simulink model "SimParking"  (R2017b)
settings: Solver=VariableStepAuto  StartTime=0.0  StopTime=1761  RelTol=1e-3
libraries: neural x1111
(part 51 of 60)

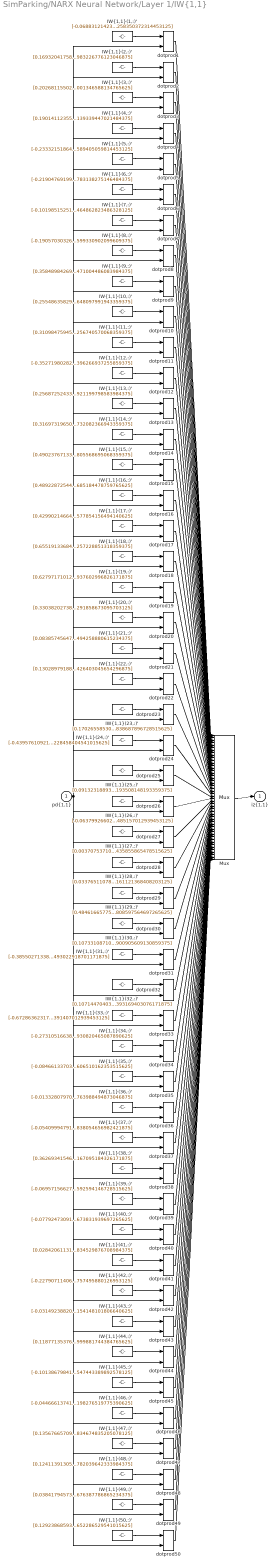
== system SimParking/NARX Neural Network/Layer 1/IW{1,1} ==
  "pd{1,1}" : Inport  PortDimensions=9  SampleTime=1
      mask Display: e = 0.06;c1 = [120 230 180]/255;c2 = ([120 230 180]+0)/(256+128);c3 = ([120 230 180]+128)/(256+128);patch([0 1 1 0],[0 0 1 1],c1);patch([0 1 1 1-e 1-e 0+e],[0 0 1 1-e 0+e 0+e],c2);patch([0 0 1 1-e 0+e 0+e],[0 1 1 1-e 1-e 0+e],c3);plot([0 1 1 0 0],[0 0 1 1 0]);
  "IW{1,1}(1,:)'" : Constant  Value=[-0.0688312142351427402875430061612860299646854400634765625;-0.00731147282474513271477434273037943057715892791748046875;0.264160400589513566504962227554642595350742340087890625;-0.2702584075688310161211802551406435668468475341796875;-0.256440287705181180211155833603697828948497772216796875;-0.032637463492422490174416083164032897911965847015380859375;0.0715212296441626038667749298838316462934017181396484375;-0.2454744006920569765473061352167860604822635650634765625;0.1741091167626269697876750797149725258350372314453125]
      mask Display: e = 0.06;c1 = [120 150 230]/255;c2 = ([120 150 230]+0)/383;c3 = ([120 150 230]+128)/383;patch([0 1 1 0],[0 0 1 1],c1);patch([0 1 1 1-e 1-e 0+e],[0 0 1 1-e 0+e 0+e],c2);patch([0 0 1 1-e 0+e 0+e],[0 1 1 1-e 1-e 0+e],c3);plot([0 1 1 0 0],[0 0 1 1 0]);disp('Weights');
  "IW{1,1}(10,:)'" : Constant  Value=[0.2554863582900424034960451535880565643310546875;0.0958506165966647449838688999079749919474124908447265625;-0.32565209786216886556076133274473249912261962890625;0.30664766510793473042184587029623799026012420654296875;0.045108980545902059577922926791870850138366222381591796875;0.13081971515873325184742270721471868455410003662109375;0.30795940572873325979941228069947101175785064697265625;0.023228248459151619453866288722565514035522937774658203125;0.2355814180893774645308980097979656420648097991943359375]
      mask Display: e = 0.06;c1 = [120 150 230]/255;c2 = ([120 150 230]+0)/383;c3 = ([120 150 230]+128)/383;patch([0 1 1 0],[0 0 1 1],c1);patch([0 1 1 1-e 1-e 0+e],[0 0 1 1-e 0+e 0+e],c2);patch([0 0 1 1-e 0+e 0+e],[0 1 1 1-e 1-e 0+e],c3);plot([0 1 1 0 0],[0 0 1 1 0]);disp('Weights');
  "IW{1,1}(11,:)'" : Constant  Value=[0.3109847594544794535664777868078090250492095947265625;-0.285941876296102959198464077417156659066677093505859375;-0.03748334600944412675627148701096302829682826995849609375;-0.4303286602511013914096338339732028543949127197265625;-0.2985573957135070344293126254342496395111083984375;0.82416954716962342875063995961681939661502838134765625;0.1697649234253264249883130787566187791526317596435546875;0.06921903233537364530381097438294091261923313140869140625;-0.27516488517038906191913838483742438256740570068359375]
      mask Display: e = 0.06;c1 = [120 150 230]/255;c2 = ([120 150 230]+0)/383;c3 = ([120 150 230]+128)/383;patch([0 1 1 0],[0 0 1 1],c1);patch([0 1 1 1-e 1-e 0+e],[0 0 1 1-e 0+e 0+e],c2);patch([0 0 1 1-e 0+e 0+e],[0 1 1 1-e 1-e 0+e],c3);plot([0 1 1 0 0],[0 0 1 1 0]);disp('Weights');
  "IW{1,1}(12,:)'" : Constant  Value=[-0.352719802824051964496021582817775197327136993408203125;-0.069499098052672791947514951971243135631084442138671875;0.3030956741440811175181124781374819576740264892578125;-0.3374792645368049903709106729365885257720947265625;0.00816585423091213853663550281680727493949234485626220703125;-0.19962942893532698018788096305797807872295379638671875;-0.20286919149293736186479009120375849306583404541015625;-0.199431767288725747544475552786025218665599822998046875;-0.345388528908461223121406646896502934396266937255859375]
      mask Display: e = 0.06;c1 = [120 150 230]/255;c2 = ([120 150 230]+0)/383;c3 = ([120 150 230]+128)/383;patch([0 1 1 0],[0 0 1 1],c1);patch([0 1 1 1-e 1-e 0+e],[0 0 1 1-e 0+e 0+e],c2);patch([0 0 1 1-e 0+e 0+e],[0 1 1 1-e 1-e 0+e],c3);plot([0 1 1 0 0],[0 0 1 1 0]);disp('Weights');
  "IW{1,1}(13,:)'" : Constant  Value=[0.256872524336901164598856439624796621501445770263671875;0.21350569072795588798641119865351356565952301025390625;-0.418804132286997532474970284965820610523223876953125;0.056591801455811004128992891537563991732895374298095703125;-0.07494113318384544586425732859424897469580173492431640625;0.2407993622761351593108969382228679023683071136474609375;0.059849568133809205594531022143200971186161041259765625;-0.060497754657408787937189487138311960734426975250244140625;0.00676880576702837931379885816340902238152921199798583984375]
      mask Display: e = 0.06;c1 = [120 150 230]/255;c2 = ([120 150 230]+0)/383;c3 = ([120 150 230]+128)/383;patch([0 1 1 0],[0 0 1 1],c1);patch([0 1 1 1-e 1-e 0+e],[0 0 1 1-e 0+e 0+e],c2);patch([0 0 1 1-e 0+e 0+e],[0 1 1 1-e 1-e 0+e],c3);plot([0 1 1 0 0],[0 0 1 1 0]);disp('Weights');
  "IW{1,1}(14,:)'" : Constant  Value=[0.316973196504036158760442276616231538355350494384765625;0.3247560829361930689884729872574098408222198486328125;0.53408347016352852865139766436186619102954864501953125;1.58975198318718202727950483676977455615997314453125;0.02759094957294229433220067448928602971136569976806640625;0.52886285187823889319957970656105317175388336181640625;0.50574814490768116304053592102718539535999298095703125;0.1567072528818204413258996510194265283644199371337890625;0.45264913068915146876491917282692156732082366943359375]
      mask Display: e = 0.06;c1 = [120 150 230]/255;c2 = ([120 150 230]+0)/383;c3 = ([120 150 230]+128)/383;patch([0 1 1 0],[0 0 1 1],c1);patch([0 1 1 1-e 1-e 0+e],[0 0 1 1-e 0+e 0+e],c2);patch([0 0 1 1-e 0+e 0+e],[0 1 1 1-e 1-e 0+e],c3);plot([0 1 1 0 0],[0 0 1 1 0]);disp('Weights');
  "IW{1,1}(15,:)'" : Constant  Value=[0.490237671330177759987378749428899027407169342041015625;0.1653204385555413491459830765961669385433197021484375;-0.79290809621698421505442411216790787875652313232421875;-0.56394479296315769278891139038023538887500762939453125;-0.01259539013756067089844226103423352469690144062042236328125;0.120847701090714354510424755062558688223361968994140625;0.11626089019634051890950132701618713326752185821533203125;0.52967211475309439183689619312644936144351959228515625;0.0275738220937100896035243380310930660925805568695068359375]
      mask Display: e = 0.06;c1 = [120 150 230]/255;c2 = ([120 150 230]+0)/383;c3 = ([120 150 230]+128)/383;patch([0 1 1 0],[0 0 1 1],c1);patch([0 1 1 1-e 1-e 0+e],[0 0 1 1-e 0+e 0+e],c2);patch([0 0 1 1-e 0+e 0+e],[0 1 1 1-e 1-e 0+e],c3);plot([0 1 1 0 0],[0 0 1 1 0]);disp('Weights');
  "IW{1,1}(16,:)'" : Constant  Value=[0.489228725449045998008301694426336325705051422119140625;-0.12693905925192827677250306805945001542568206787109375;0.1444743099035981914735060627208440564572811126708984375;0.43394957527358801741002025664784014225006103515625;0.1301043144415301444638544126064516603946685791015625;0.185288074364715560360394874805933795869350433349609375;0.3632901734391797976542193282512016594409942626953125;0.272778700473264190673461371261510066688060760498046875;0.0155539985865831321965035982657354907132685184478759765625]
      mask Display: e = 0.06;c1 = [120 150 230]/255;c2 = ([120 150 230]+0)/383;c3 = ([120 150 230]+128)/383;patch([0 1 1 0],[0 0 1 1],c1);patch([0 1 1 1-e 1-e 0+e],[0 0 1 1-e 0+e 0+e],c2);patch([0 0 1 1-e 0+e 0+e],[0 1 1 1-e 1-e 0+e],c3);plot([0 1 1 0 0],[0 0 1 1 0]);disp('Weights');
  "IW{1,1}(17,:)'" : Constant  Value=[0.429902146643838689588079660097719170153141021728515625;0.257765727905190866753315503956400789320468902587890625;-0.1500747886843795397826539783636690117418766021728515625;0.278788719014294417153365657213726080954074859619140625;0.276750512007699234207080962733016349375247955322265625;-0.82138062848648729641354293562471866607666015625;0.27536313592640848657566721158218570053577423095703125;0.1430395985820490933893012197586358524858951568603515625;0.348188489253207722473604235347011126577854156494140625]
      mask Display: e = 0.06;c1 = [120 150 230]/255;c2 = ([120 150 230]+0)/383;c3 = ([120 150 230]+128)/383;patch([0 1 1 0],[0 0 1 1],c1);patch([0 1 1 1-e 1-e 0+e],[0 0 1 1-e 0+e 0+e],c2);patch([0 0 1 1-e 0+e 0+e],[0 1 1 1-e 1-e 0+e],c3);plot([0 1 1 0 0],[0 0 1 1 0]);disp('Weights');
  "IW{1,1}(18,:)'" : Constant  Value=[0.65519133684555008745320492380415089428424835205078125;-0.456854910966180527420732460086583159863948822021484375;1.3571548324974906929440976455225609242916107177734375;0.34003096030817392403378107701428234577178955078125;-0.29173479660044321359890773237566463649272918701171875;0.376176211592635867386746895135729573667049407958984375;0.234861025309017090734187149791978299617767333984375;0.320971922147644417311340703236055560410022735595703125;0.1188667057288495809697081995182088576257228851318359375]
      mask Display: e = 0.06;c1 = [120 150 230]/255;c2 = ([120 150 230]+0)/383;c3 = ([120 150 230]+128)/383;patch([0 1 1 0],[0 0 1 1],c1);patch([0 1 1 1-e 1-e 0+e],[0 0 1 1-e 0+e 0+e],c2);patch([0 0 1 1-e 0+e 0+e],[0 1 1 1-e 1-e 0+e],c3);plot([0 1 1 0 0],[0 0 1 1 0]);disp('Weights');
  "IW{1,1}(19,:)'" : Constant  Value=[0.6279717101208761587116669034003280103206634521484375;-0.215597262533756051094968597681145183742046356201171875;-0.62907101345034532879907374081085436046123504638671875;-0.495109753658072804238798880760441534221172332763671875;-0.05778022558784827455991006672775256447494029998779296875;-1.0225979740194868217173507218831218779087066650390625;-0.03403932971557062370226987013666075654327869415283203125;-0.30098566072865640119715635592001490294933319091796875;-0.0220281334301075486237220246721335570327937602996826171875]
      mask Display: e = 0.06;c1 = [120 150 230]/255;c2 = ([120 150 230]+0)/383;c3 = ([120 150 230]+128)/383;patch([0 1 1 0],[0 0 1 1],c1);patch([0 1 1 1-e 1-e 0+e],[0 0 1 1-e 0+e 0+e],c2);patch([0 0 1 1-e 0+e 0+e],[0 1 1 1-e 1-e 0+e],c3);plot([0 1 1 0 0],[0 0 1 1 0]);disp('Weights');
  "IW{1,1}(2,:)'" : Constant  Value=[0.1693204175805965994161539356355206109583377838134765625;-0.280434391905482416351702568135806359350681304931640625;0.5574414461071182103069077129475772380828857421875;0.1491102386444250471608796715372591279447078704833984375;-0.139621185316120388630878323965589515864849090576171875;0.413097455057599594052675229249871335923671722412109375;-0.0987573011740672523917083935884875245392322540283203125;0.285585829665227441953589959666715003550052642822265625;0.09414021440129786977291104221876594237983226776123046875]
      mask Display: e = 0.06;c1 = [120 150 230]/255;c2 = ([120 150 230]+0)/383;c3 = ([120 150 230]+128)/383;patch([0 1 1 0],[0 0 1 1],c1);patch([0 1 1 1-e 1-e 0+e],[0 0 1 1-e 0+e 0+e],c2);patch([0 0 1 1-e 0+e 0+e],[0 1 1 1-e 1-e 0+e],c3);plot([0 1 1 0 0],[0 0 1 1 0]);disp('Weights');
  "IW{1,1}(20,:)'" : Constant  Value=[0.3303820273860218481587480710004456341266632080078125;0.042681097483308734485962787630342063494026660919189453125;-4.19220558490714179100677938549779355525970458984375;-2.64104506999998900340642649098299443721771240234375;0.124710532719106648169571371909114532172679901123046875;-0.20265695712461428978912181264604441821575164794921875;0.2237739206169422623293741025918279774487018585205078125;0.263060219041964693520441187502001412212848663330078125;0.72859097760744984118019829111290164291858673095703125]
      mask Display: e = 0.06;c1 = [120 150 230]/255;c2 = ([120 150 230]+0)/383;c3 = ([120 150 230]+128)/383;patch([0 1 1 0],[0 0 1 1],c1);patch([0 1 1 1-e 1-e 0+e],[0 0 1 1-e 0+e 0+e],c2);patch([0 0 1 1-e 0+e 0+e],[0 1 1 1-e 1-e 0+e],c3);plot([0 1 1 0 0],[0 0 1 1 0]);disp('Weights');
  "IW{1,1}(21,:)'" : Constant  Value=[0.08385745647819399517519656228614621795713901519775390625;-0.497456497766189775777689874303177930414676666259765625;1.0492079261781894761185185416252352297306060791015625;-0.1906673066428924145920831278999685309827327728271484375;-0.171599694156398030475685345663805492222309112548828125;-0.360786631499553533952706629861495457589626312255859375;-0.0961295972527534126061965480403159745037555694580078125;-0.298552069183902257787366352204116992652416229248046875;-0.007428480862369322111626868121447841986082494258880615234375]
      mask Display: e = 0.06;c1 = [120 150 230]/255;c2 = ([120 150 230]+0)/383;c3 = ([120 150 230]+128)/383;patch([0 1 1 0],[0 0 1 1],c1);patch([0 1 1 1-e 1-e 0+e],[0 0 1 1-e 0+e 0+e],c2);patch([0 0 1 1-e 0+e 0+e],[0 1 1 1-e 1-e 0+e],c3);plot([0 1 1 0 0],[0 0 1 1 0]);disp('Weights');
  "IW{1,1}(22,:)'" : Constant  Value=[0.130289791885517092229207491982378996908664703369140625;0.1800086656054050437969493714263080619275569915771484375;-0.49670794016582331398268479460966773331165313720703125;0.292715502828505391708091565305949188768863677978515625;0.2950565389889596712436059533501975238323211669921875;-0.7203712354727842548385297050117515027523040771484375;-0.1973878324567578113057919608763768337666988372802734375;0.1061907764516101526641733698852476663887500762939453125;0.08327945591651368661967325124351191334426403045654296875]
      mask Display: e = 0.06;c1 = [120 150 230]/255;c2 = ([120 150 230]+0)/383;c3 = ([120 150 230]+128)/383;patch([0 1 1 0],[0 0 1 1],c1);patch([0 1 1 1-e 1-e 0+e],[0 0 1 1-e 0+e 0+e],c2);patch([0 0 1 1-e 0+e 0+e],[0 1 1 1-e 1-e 0+e],c3);plot([0 1 1 0 0],[0 0 1 1 0]);disp('Weights');
  "IW{1,1}(23,:)'" : Constant  Value=[0.170265585301424160480365799230639822781085968017578125;0.0017600261592727304595096260442232960485853254795074462890625;0.15747452750562340728635035702609457075595855712890625;-0.496485958274373195830975191711331717669963836669921875;0.037768686613442355171077480235908296890556812286376953125;-0.6705335286781721748639029101468622684478759765625;-0.57073263733206081038673573857522569596767425537109375;-0.2755979057809099241893591170082800090312957763671875;-0.375640180372313337020528933862806297838687896728515625]
      mask Display: e = 0.06;c1 = [120 150 230]/255;c2 = ([120 150 230]+0)/383;c3 = ([120 150 230]+128)/383;patch([0 1 1 0],[0 0 1 1],c1);patch([0 1 1 1-e 1-e 0+e],[0 0 1 1-e 0+e 0+e],c2);patch([0 0 1 1-e 0+e 0+e],[0 1 1 1-e 1-e 0+e],c3);plot([0 1 1 0 0],[0 0 1 1 0]);disp('Weights');
  "IW{1,1}(24,:)'" : Constant  Value=[-0.439576109215813970454433956547291018068790435791015625;-0.2189663763544104357894326540190377272665500640869140625;0.2475990245909240050625754747670725919306278228759765625;0.001023972132195846880542422496773724560625851154327392578125;0.0219517589493653970944553321942294132895767688751220703125;-0.2427449940657558646872615781830972991883754730224609375;0.04118883159793640391654889754136092960834503173828125;-0.1600808104926337571694006101097329519689083099365234375;-0.009550439179479099094383087731330306269228458404541015625]
      mask Display: e = 0.06;c1 = [120 150 230]/255;c2 = ([120 150 230]+0)/383;c3 = ([120 150 230]+128)/383;patch([0 1 1 0],[0 0 1 1],c1);patch([0 1 1 1-e 1-e 0+e],[0 0 1 1-e 0+e 0+e],c2);patch([0 0 1 1-e 0+e 0+e],[0 1 1 1-e 1-e 0+e],c3);plot([0 1 1 0 0],[0 0 1 1 0]);disp('Weights');
  "IW{1,1}(25,:)'" : Constant  Value=[0.09132318893893198730182803046773187816143035888671875;-0.305736356371004325271911739037022925913333892822265625;0.2135115652303083699781183213417534716427326202392578125;0.230298438032124630492347705512656830251216888427734375;0.2103100040246245472363995077103027142584323883056640625;0.1845883825576032088999767211134894751012325286865234375;0.2075026611736426052079451665122178383171558380126953125;0.103496987083271096974357305953162722289562225341796875;0.198160953523112137730777249089442193508148193359375]
      mask Display: e = 0.06;c1 = [120 150 230]/255;c2 = ([120 150 230]+0)/383;c3 = ([120 150 230]+128)/383;patch([0 1 1 0],[0 0 1 1],c1);patch([0 1 1 1-e 1-e 0+e],[0 0 1 1-e 0+e 0+e],c2);patch([0 0 1 1-e 0+e 0+e],[0 1 1 1-e 1-e 0+e],c3);plot([0 1 1 0 0],[0 0 1 1 0]);disp('Weights');
  "IW{1,1}(26,:)'" : Constant  Value=[-0.063799266029572976322015165351331233978271484375;-0.10732348297887218946389253915185690857470035552978515625;0.42759446964219038900267833014368079602718353271484375;0.49455718016339444975670858184457756578922271728515625;0.06096643228676323911230383600923232734203338623046875;-0.50868524934939518544751990702934563159942626953125;-0.310900507489883570766409093266702257096767425537109375;0.254270372723495674538440880496636964380741119384765625;0.437813272126399699590848513253149576485157012939453125]
      mask Display: e = 0.06;c1 = [120 150 230]/255;c2 = ([120 150 230]+0)/383;c3 = ([120 150 230]+128)/383;patch([0 1 1 0],[0 0 1 1],c1);patch([0 1 1 1-e 1-e 0+e],[0 0 1 1-e 0+e 0+e],c2);patch([0 0 1 1-e 0+e 0+e],[0 1 1 1-e 1-e 0+e],c3);plot([0 1 1 0 0],[0 0 1 1 0]);disp('Weights');
  "IW{1,1}(27,:)'" : Constant  Value=[0.0037075371066769753115865970727327294298447668552398681640625;-0.0472743800535389280259579436460626311600208282470703125;1.5418866471201189138895415453589521348476409912109375;0.82584125802911934055572373836184851825237274169921875;0.1409274956894774055715657823384390212595462799072265625;-0.32051144913274765002597632701508700847625732421875;0.060628886477887521111451718525131582282483577728271484375;0.148480475088179797449328134462120942771434783935546875;-0.54728493235290598395437200451851822435855865478515625]
      mask Display: e = 0.06;c1 = [120 150 230]/255;c2 = ([120 150 230]+0)/383;c3 = ([120 150 230]+128)/383;patch([0 1 1 0],[0 0 1 1],c1);patch([0 1 1 1-e 1-e 0+e],[0 0 1 1-e 0+e 0+e],c2);patch([0 0 1 1-e 0+e 0+e],[0 1 1 1-e 1-e 0+e],c3);plot([0 1 1 0 0],[0 0 1 1 0]);disp('Weights');
  "IW{1,1}(28,:)'" : Constant  Value=[0.033765110786281839205802413061974220909178256988525390625;-0.26436983167133398797687959813629277050495147705078125;-0.465795196418422874362619268140406347811222076416015625;-0.338173945717743673622379674270632676780223846435546875;-0.149619516236496885586149119262699969112873077392578125;0.0176859274169523759956401676163295633159577846527099609375;-0.70075171210961528789340491130133159458637237548828125;-0.1497602357242875104059720570148783735930919647216796875;-0.64481354172627913801107979452353902161121368408203125]
      mask Display: e = 0.06;c1 = [120 150 230]/255;c2 = ([120 150 230]+0)/383;c3 = ([120 150 230]+128)/383;patch([0 1 1 0],[0 0 1 1],c1);patch([0 1 1 1-e 1-e 0+e],[0 0 1 1-e 0+e 0+e],c2);patch([0 0 1 1-e 0+e 0+e],[0 1 1 1-e 1-e 0+e],c3);plot([0 1 1 0 0],[0 0 1 1 0]);disp('Weights');
  "IW{1,1}(29,:)'" : Constant  Value=[0.4846166577505750527876671185367740690708160400390625;0.0287723940911300650469240025586259434930980205535888671875;0.39182719001120547286376449847011826932430267333984375;-0.036557942285625470713039675274558248929679393768310546875;-0.157521689983647739108363339255447499454021453857421875;-1.5927902688797501706829962131450884044170379638671875;-0.26962413257348571971050432694028131663799285888671875;-0.10568969672952821525768740684725344181060791015625;0.478447962415805339020380415604449808597564697265625]
      mask Display: e = 0.06;c1 = [120 150 230]/255;c2 = ([120 150 230]+0)/383;c3 = ([120 150 230]+128)/383;patch([0 1 1 0],[0 0 1 1],c1);patch([0 1 1 1-e 1-e 0+e],[0 0 1 1-e 0+e 0+e],c2);patch([0 0 1 1-e 0+e 0+e],[0 1 1 1-e 1-e 0+e],c3);plot([0 1 1 0 0],[0 0 1 1 0]);disp('Weights');
  "IW{1,1}(3,:)'" : Constant  Value=[0.2026811550245939119729854382967459969222545623779296875;-0.00984209151891591270400194702006047009490430355072021484375;-0.1392976250777042401818306416316772811114788055419921875;0.2836347563671746119240424377494491636753082275390625;0.171277805649655723296831411062157712876796722412109375;0.4053455908656935502420992634142749011516571044921875;-0.154302720015346894744112660191603936254978179931640625;0.0059490774025495463117607641834183596074581146240234375;-0.382239825931924903645864333157078363001346588134765625]
      mask Display: e = 0.06;c1 = [120 150 230]/255;c2 = ([120 150 230]+0)/383;c3 = ([120 150 230]+128)/383;patch([0 1 1 0],[0 0 1 1],c1);patch([0 1 1 1-e 1-e 0+e],[0 0 1 1-e 0+e 0+e],c2);patch([0 0 1 1-e 0+e 0+e],[0 1 1 1-e 1-e 0+e],c3);plot([0 1 1 0 0],[0 0 1 1 0]);disp('Weights');
  "IW{1,1}(30,:)'" : Constant  Value=[0.1073310871065546734381968008165131323039531707763671875;-5.73810811118678309843132989698233359376899898052215576171875e-05;-0.1779937377257815034337085080551332794129848480224609375;0.1285949133065027172317940085122245363891124725341796875;-0.0805135342172788870396260563211399130523204803466796875;0.389025764725511369324095767296967096626758575439453125;0.1899070574171372316474304398070671595633029937744140625;0.1915964846254201436881459130745497532188892364501953125;0.01273686929292105161903858601135652861557900905609130859375]
      mask Display: e = 0.06;c1 = [120 150 230]/255;c2 = ([120 150 230]+0)/383;c3 = ([120 150 230]+128)/383;patch([0 1 1 0],[0 0 1 1],c1);patch([0 1 1 1-e 1-e 0+e],[0 0 1 1-e 0+e 0+e],c2);patch([0 0 1 1-e 0+e 0+e],[0 1 1 1-e 1-e 0+e],c3);plot([0 1 1 0 0],[0 0 1 1 0]);disp('Weights');
  "IW{1,1}(31,:)'" : Constant  Value=[-0.385502713380549477673042702008388005197048187255859375;0.021935718119657283964318850166819174773991107940673828125;-1.1925166228482932950782924308441579341888427734375;0.0575735896712597228219721046116319485008716583251953125;0.08673079327070742916561130186892114579677581787109375;0.9971501246260381368102798660402186214923858642578125;0.04098675601681965596778667304533882997930049896240234375;0.2483047315550218903101864498239592649042606353759765625;-0.034756059840693347140483382418096880428493022918701171875]
      mask Display: e = 0.06;c1 = [120 150 230]/255;c2 = ([120 150 230]+0)/383;c3 = ([120 150 230]+128)/383;patch([0 1 1 0],[0 0 1 1],c1);patch([0 1 1 1-e 1-e 0+e],[0 0 1 1-e 0+e 0+e],c2);patch([0 0 1 1-e 0+e 0+e],[0 1 1 1-e 1-e 0+e],c3);plot([0 1 1 0 0],[0 0 1 1 0]);disp('Weights');
  "IW{1,1}(32,:)'" : Constant  Value=[0.1071447040357628444073867512997821904718875885009765625;0.224815387460384263906831847634748555719852447509765625;-0.53466918219139769608005963164032436907291412353515625;-0.1738107812905509141909732306885416619479656219482421875;0.304319718206822964479130178006016649305820465087890625;0.01730921322648147631095838505643769167363643646240234375;-0.171529915698019175263056013136520050466060638427734375;0.093775137038517086818245616086642257869243621826171875;0.10215241716838723007310107959710876457393169403076171875]
      mask Display: e = 0.06;c1 = [120 150 230]/255;c2 = ([120 150 230]+0)/383;c3 = ([120 150 230]+128)/383;patch([0 1 1 0],[0 0 1 1],c1);patch([0 1 1 1-e 1-e 0+e],[0 0 1 1-e 0+e 0+e],c2);patch([0 0 1 1-e 0+e 0+e],[0 1 1 1-e 1-e 0+e],c3);plot([0 1 1 0 0],[0 0 1 1 0]);disp('Weights');
  "IW{1,1}(33,:)'" : Constant  Value=[-0.6728636231709692605562622702564112842082977294921875;0.340403461100505622116685344735742546617984771728515625;0.49412251624778746883492885899613611400127410888671875;1.0153357855302289625143430384923703968524932861328125;-0.127101222003216329792252281549735926091670989990234375;-0.034716665267675646255884913671252434141933917999267578125;1.066642997710553597556781824096105992794036865234375;0.52895280866874594405402376651181839406490325927734375;0.32620825228680150331683762487955391407012939453125]
      mask Display: e = 0.06;c1 = [120 150 230]/255;c2 = ([120 150 230]+0)/383;c3 = ([120 150 230]+128)/383;patch([0 1 1 0],[0 0 1 1],c1);patch([0 1 1 1-e 1-e 0+e],[0 0 1 1-e 0+e 0+e],c2);patch([0 0 1 1-e 0+e 0+e],[0 1 1 1-e 1-e 0+e],c3);plot([0 1 1 0 0],[0 0 1 1 0]);disp('Weights');
  "IW{1,1}(34,:)'" : Constant  Value=[-0.2731051663864632050859881928772665560245513916015625;-0.28488050080682558728994990815408527851104736328125;0.39631433764840784395033779219374991953372955322265625;-0.38869351408481078724577173488796688616275787353515625;0.0158544792163410573626602939611984766088426113128662109375;-0.31241314724041246986274700248031876981258392333984375;-0.0175040717768346655580646853422877029515802860260009765625;-0.302997522510356553926413880617474205791950225830078125;0.1711228322823369618621569543392979539930820465087890625]
      mask Display: e = 0.06;c1 = [120 150 230]/255;c2 = ([120 150 230]+0)/383;c3 = ([120 150 230]+128)/383;patch([0 1 1 0],[0 0 1 1],c1);patch([0 1 1 1-e 1-e 0+e],[0 0 1 1-e 0+e 0+e],c2);patch([0 0 1 1-e 0+e 0+e],[0 1 1 1-e 1-e 0+e],c3);plot([0 1 1 0 0],[0 0 1 1 0]);disp('Weights');
  "IW{1,1}(35,:)'" : Constant  Value=[-0.084661337035410400009283193867304362356662750244140625;-0.1401330260330958255021727154598920606076717376708984375;0.92347381064149314244815514030051417648792266845703125;1.1165443472979654782051284200861118733882904052734375;-0.167030675953085239182627219634014181792736053466796875;-0.249815597775006781322559845648356713354587554931640625;-0.08475732918876517640871526282353443093597888946533203125;-0.426932020655221844407378739560954272747039794921875;-1.1807403748280320687769062715233303606510162353515625]
      mask Display: e = 0.06;c1 = [120 150 230]/255;c2 = ([120 150 230]+0)/383;c3 = ([120 150 230]+128)/383;patch([0 1 1 0],[0 0 1 1],c1);patch([0 1 1 1-e 1-e 0+e],[0 0 1 1-e 0+e 0+e],c2);patch([0 0 1 1-e 0+e 0+e],[0 1 1 1-e 1-e 0+e],c3);plot([0 1 1 0 0],[0 0 1 1 0]);disp('Weights');
  "IW{1,1}(36,:)'" : Constant  Value=[-0.01332807970061637529990417050385076436214148998260498046875;0.1502274065987534712451889618023415096104145050048828125;0.148524573999566700255314799505867995321750640869140625;0.2478074239673170586772954493426368571817874908447265625;0.006483220831589870357392069166735382168553769588470458984375;0.420228421724278933258034385289647616446018218994140625;0.08812894848820114479526210971016553230583667755126953125;-0.07764713089344198182484291237415163777768611907958984375;0.09461569659726258574306001492004725150763988494873046875]
      mask Display: e = 0.06;c1 = [120 150 230]/255;c2 = ([120 150 230]+0)/383;c3 = ([120 150 230]+128)/383;patch([0 1 1 0],[0 0 1 1],c1);patch([0 1 1 1-e 1-e 0+e],[0 0 1 1-e 0+e 0+e],c2);patch([0 0 1 1-e 0+e 0+e],[0 1 1 1-e 1-e 0+e],c3);plot([0 1 1 0 0],[0 0 1 1 0]);disp('Weights');
  "IW{1,1}(37,:)'" : Constant  Value=[-0.054099947911962674440555787214179872535169124603271484375;0.032532056899680840411637205988881760276854038238525390625;0.178141170473542442831416110493591986596584320068359375;-0.4085330283853274568883762185578234493732452392578125;-0.01858464167620989260232278184048482216894626617431640625;-0.209578183565288067580212327811750583350658416748046875;-0.1003992996928394776379178665592917241156101226806640625;0.01185436983745245635712972642750173690728843212127685546875;-0.08261153730344998613599472037094528786838054656982421875]
      mask Display: e = 0.06;c1 = [120 150 230]/255;c2 = ([120 150 230]+0)/383;c3 = ([120 150 230]+128)/383;patch([0 1 1 0],[0 0 1 1],c1);patch([0 1 1 1-e 1-e 0+e],[0 0 1 1-e 0+e 0+e],c2);patch([0 0 1 1-e 0+e 0+e],[0 1 1 1-e 1-e 0+e],c3);plot([0 1 1 0 0],[0 0 1 1 0]);disp('Weights');
  "IW{1,1}(38,:)'" : Constant  Value=[0.36269341546568634182534651699825190007686614990234375;0.15810102266780001745161143844597972929477691650390625;0.1260473858878371211655888828317984007298946380615234375;-0.140919489927845364984904108496266417205333709716796875;-0.2578969885013133733764334465377032756805419921875;0.89179668107359078010887287746299989521503448486328125;0.260908402651786219816898437784402631223201751708984375;-0.033687070002127901535704523894310113973915576934814453125;0.07039178526726712348260406315603177063167095184326171875]
      mask Display: e = 0.06;c1 = [120 150 230]/255;c2 = ([120 150 230]+0)/383;c3 = ([120 150 230]+128)/383;patch([0 1 1 0],[0 0 1 1],c1);patch([0 1 1 1-e 1-e 0+e],[0 0 1 1-e 0+e 0+e],c2);patch([0 0 1 1-e 0+e 0+e],[0 1 1 1-e 1-e 0+e],c3);plot([0 1 1 0 0],[0 0 1 1 0]);disp('Weights');
  "IW{1,1}(39,:)'" : Constant  Value=[-0.0695715662777189047805137533941888250410556793212890625;-0.0872057719177930235066042996550095267593860626220703125;0.0952131614734814391010075951271574012935161590576171875;0.00840796137645711573471718480732306488789618015289306640625;0.022793649555518789850960814646896324120461940765380859375;-0.254842509595828825563756936389836482703685760498046875;-0.17833154015167174133438265926088206470012664794921875;0.08100298512418903362775068899281905032694339752197265625;-0.204522709085990739286131656626821495592594146728515625]
      mask Display: e = 0.06;c1 = [120 150 230]/255;c2 = ([120 150 230]+0)/383;c3 = ([120 150 230]+128)/383;patch([0 1 1 0],[0 0 1 1],c1);patch([0 1 1 1-e 1-e 0+e],[0 0 1 1-e 0+e 0+e],c2);patch([0 0 1 1-e 0+e 0+e],[0 1 1 1-e 1-e 0+e],c3);plot([0 1 1 0 0],[0 0 1 1 0]);disp('Weights');
  "IW{1,1}(4,:)'" : Constant  Value=[0.1901411235583422010275711500071338377892971038818359375;-0.1801140604737041517324769301922060549259185791015625;0.43908829385588343807711453337105922400951385498046875;0.300742867669990310286465273748035542666912078857421875;-0.261778202961331529774469117910484783351421356201171875;0.0011562680449718385454482838525791521533392369747161865234375;0.14908281020036218134094951892620883882045745849609375;0.1642118843967598496025317444946267642080783843994140625;-0.11180962823186556265309121727113961242139339447021484375]
      mask Display: e = 0.06;c1 = [120 150 230]/255;c2 = ([120 150 230]+0)/383;c3 = ([120 150 230]+128)/383;patch([0 1 1 0],[0 0 1 1],c1);patch([0 1 1 1-e 1-e 0+e],[0 0 1 1-e 0+e 0+e],c2);patch([0 0 1 1-e 0+e 0+e],[0 1 1 1-e 1-e 0+e],c3);plot([0 1 1 0 0],[0 0 1 1 0]);disp('Weights');
  "IW{1,1}(40,:)'" : Constant  Value=[-0.07792473091857965439288591369404457509517669677734375;0.12262579073976458132744227214061538688838481903076171875;0.433585751238178662703148802393116056919097900390625;0.4483744159696907427559153802576474845409393310546875;-0.0909994008640116203157077734431368298828601837158203125;0.1909432868732878763040616831858642399311065673828125;0.4665394114890906163140016360557638108730316162109375;0.018369676388352067231135578140310826711356639862060546875;-0.36320516690140414173271210529492236673831939697265625]
      mask Display: e = 0.06;c1 = [120 150 230]/255;c2 = ([120 150 230]+0)/383;c3 = ([120 150 230]+128)/383;patch([0 1 1 0],[0 0 1 1],c1);patch([0 1 1 1-e 1-e 0+e],[0 0 1 1-e 0+e 0+e],c2);patch([0 0 1 1-e 0+e 0+e],[0 1 1 1-e 1-e 0+e],c3);plot([0 1 1 0 0],[0 0 1 1 0]);disp('Weights');
  "IW{1,1}(41,:)'" : Constant  Value=[0.028420611312396489023246459737492841668426990509033203125;-0.19039724289141923829760116859688423573970794677734375;0.1965215276589629411763127109225024469196796417236328125;0.2247339932238971715872111190037685446441173553466796875;0.250863124992955210945666522093233652412891387939453125;-0.06694716420891345942667527424418949522078037261962890625;-0.0103644737274374738877913415535658714361488819122314453125;0.1639503748178644249033908408819115720689296722412109375;0.08990803987677629949271107534514158032834529876708984375]
      mask Display: e = 0.06;c1 = [120 150 230]/255;c2 = ([120 150 230]+0)/383;c3 = ([120 150 230]+128)/383;patch([0 1 1 0],[0 0 1 1],c1);patch([0 1 1 1-e 1-e 0+e],[0 0 1 1-e 0+e 0+e],c2);patch([0 0 1 1-e 0+e 0+e],[0 1 1 1-e 1-e 0+e],c3);plot([0 1 1 0 0],[0 0 1 1 0]);disp('Weights');
  "IW{1,1}(42,:)'" : Constant  Value=[-0.227907114060305782121673701112740673124790191650390625;0.0529159160157012531389142395710223354399204254150390625;0.38495511040741536845644077402539551258087158203125;0.07055459584924390903371005379085545428097248077392578125;0.1225403963357225567420982770272530615329742431640625;0.270848052832142582868613089885911904275417327880859375;0.063806971941492485189684202850912697613239288330078125;0.376760359425911850461687890856410376727581024169921875;0.054719370688788522560930260851819184608757495880126953125]
      mask Display: e = 0.06;c1 = [120 150 230]/255;c2 = ([120 150 230]+0)/383;c3 = ([120 150 230]+128)/383;patch([0 1 1 0],[0 0 1 1],c1);patch([0 1 1 1-e 1-e 0+e],[0 0 1 1-e 0+e 0+e],c2);patch([0 0 1 1-e 0+e 0+e],[0 1 1 1-e 1-e 0+e],c3);plot([0 1 1 0 0],[0 0 1 1 0]);disp('Weights');
  "IW{1,1}(43,:)'" : Constant  Value=[-0.03149238820964987695116832355779479257762432098388671875;0.10050043322096972875367981714589404873549938201904296875;-0.2013123762112749293162750063856947235763072967529296875;-0.3296639854323319962503546776133589446544647216796875;0.039504122430972725410480705932059208862483501434326171875;-1.09238157279437064772764642839320003986358642578125;-0.07196411568650400158997371136138099245727062225341796875;0.08868413464713721661158984943540417589247226715087890625;-0.31838953259205171608670070781954564154148101806640625]
      mask Display: e = 0.06;c1 = [120 150 230]/255;c2 = ([120 150 230]+0)/383;c3 = ([120 150 230]+128)/383;patch([0 1 1 0],[0 0 1 1],c1);patch([0 1 1 1-e 1-e 0+e],[0 0 1 1-e 0+e 0+e],c2);patch([0 0 1 1-e 0+e 0+e],[0 1 1 1-e 1-e 0+e],c3);plot([0 1 1 0 0],[0 0 1 1 0]);disp('Weights');
  "IW{1,1}(44,:)'" : Constant  Value=[0.11877135376971224844933061604024260304868221282958984375;0.115605196373715635171919302592868916690349578857421875;-0.332338091469648322373586779576726257801055908203125;0.41114608845836031481013606025953777134418487548828125;0.07383493238482785603338243163307197391986846923828125;-0.1470944228292858368956075310052256099879741668701171875;0.090888381054905653666509124377625994384288787841796875;0.0929387258775238311869770768680609762668609619140625;0.28193331659010445466861938257352448999881744384765625]
      mask Display: e = 0.06;c1 = [120 150 230]/255;c2 = ([120 150 230]+0)/383;c3 = ([120 150 230]+128)/383;patch([0 1 1 0],[0 0 1 1],c1);patch([0 1 1 1-e 1-e 0+e],[0 0 1 1-e 0+e 0+e],c2);patch([0 0 1 1-e 0+e 0+e],[0 1 1 1-e 1-e 0+e],c3);plot([0 1 1 0 0],[0 0 1 1 0]);disp('Weights');
  "IW{1,1}(45,:)'" : Constant  Value=[-0.10138679841559457284194678550193202681839466094970703125;-0.003503666147639562800097934314180747605860233306884765625;-0.106974894713981638627586789880297146737575531005859375;-0.0915626330787251418996675056405365467071533203125;-0.266613716648214704729724644494126550853252410888671875;-0.31348596250773297366976066768984310328960418701171875;-0.0169652202903525749222435337060232996009290218353271484375;-0.1990672543813097050691141021161456592381000518798828125;-0.1762107111909678724970262919669039547443389892578125]
      mask Display: e = 0.06;c1 = [120 150 230]/255;c2 = ([120 150 230]+0)/383;c3 = ([120 150 230]+128)/383;patch([0 1 1 0],[0 0 1 1],c1);patch([0 1 1 1-e 1-e 0+e],[0 0 1 1-e 0+e 0+e],c2);patch([0 0 1 1-e 0+e 0+e],[0 1 1 1-e 1-e 0+e],c3);plot([0 1 1 0 0],[0 0 1 1 0]);disp('Weights');
  "IW{1,1}(46,:)'" : Constant  Value=[-0.044666137418643579726218462155884481035172939300537109375;0.2166254145504493688889624536386691033840179443359375;-0.04672716595910265946489658972495817579329013824462890625;-0.02552469453907275920290231852050055749714374542236328125;0.239627223619819862410196265045669861137866973876953125;-0.11765685573425262167024385462354985065758228302001953125;-0.00370282972631650643402512201873832964338362216949462890625;0.1319313165876540294707552902764291502535343170166015625;0.26040734001040244383062827182584442198276519775390625]
      mask Display: e = 0.06;c1 = [120 150 230]/255;c2 = ([120 150 230]+0)/383;c3 = ([120 150 230]+128)/383;patch([0 1 1 0],[0 0 1 1],c1);patch([0 1 1 1-e 1-e 0+e],[0 0 1 1-e 0+e 0+e],c2);patch([0 0 1 1-e 0+e 0+e],[0 1 1 1-e 1-e 0+e],c3);plot([0 1 1 0 0],[0 0 1 1 0]);disp('Weights');
  "IW{1,1}(47,:)'" : Constant  Value=[0.135676657096902186783182742146891541779041290283203125;0.21050470261408771310840393198304809629917144775390625;-0.4640822861016957734392462953110225498676300048828125;0.306659201255361557603151823059306479990482330322265625;0.08148985934319379065282618057608488015830516815185546875;0.246440662308831714977230831209453754127025604248046875;-0.0154729336182477632266607514566203462891280651092529296875;0.1356651296414167207071699294829159043729305267333984375;0.2051554500540149483800433927171980030834674835205078125]
      mask Display: e = 0.06;c1 = [120 150 230]/255;c2 = ([120 150 230]+0)/383;c3 = ([120 150 230]+128)/383;patch([0 1 1 0],[0 0 1 1],c1);patch([0 1 1 1-e 1-e 0+e],[0 0 1 1-e 0+e 0+e],c2);patch([0 0 1 1-e 0+e 0+e],[0 1 1 1-e 1-e 0+e],c3);plot([0 1 1 0 0],[0 0 1 1 0]);disp('Weights');
  "IW{1,1}(48,:)'" : Constant  Value=[0.12411391305348555558207834792483481578528881072998046875;-0.045080733615394490143568617668279330246150493621826171875;0.291180061270856771482584690602379851043224334716796875;-0.051756234289968304496110107493223040364682674407958984375;-0.185892488303269043381504843637230806052684783935546875;0.1483322318417769347664858514690422452986240386962890625;0.05894183553817329557222848279707250185310840606689453125;0.23401871568549947877357908510020934045314788818359375;0.258951333208738476709953602039604447782039642333984375]
      mask Display: e = 0.06;c1 = [120 150 230]/255;c2 = ([120 150 230]+0)/383;c3 = ([120 150 230]+128)/383;patch([0 1 1 0],[0 0 1 1],c1);patch([0 1 1 1-e 1-e 0+e],[0 0 1 1-e 0+e 0+e],c2);patch([0 0 1 1-e 0+e 0+e],[0 1 1 1-e 1-e 0+e],c3);plot([0 1 1 0 0],[0 0 1 1 0]);disp('Weights');
  "IW{1,1}(49,:)'" : Constant  Value=[0.038417945731955983890149042281336733140051364898681640625;-0.01824237752665579248567695458405069075524806976318359375;0.43965906381517949608195294786128215491771697998046875;0.204718183541127085600663804143550805747509002685546875;0.0790864264686692575168081020819954574108123779296875;0.55198238322071901951204608849366195499897003173828125;0.024919173210657320771677092352547333575785160064697265625;0.0266804726395297835128683772154545295052230358123779296875;-0.10044018647099726970761679467614158056676387786865234375]
      mask Display: e = 0.06;c1 = [120 150 230]/255;c2 = ([120 150 230]+0)/383;c3 = ([120 150 230]+128)/383;patch([0 1 1 0],[0 0 1 1],c1);patch([0 1 1 1-e 1-e 0+e],[0 0 1 1-e 0+e 0+e],c2);patch([0 0 1 1-e 0+e 0+e],[0 1 1 1-e 1-e 0+e],c3);plot([0 1 1 0 0],[0 0 1 1 0]);disp('Weights');
  "IW{1,1}(5,:)'" : Constant  Value=[-0.2333215186449786038291875911454553715884685516357421875;-0.1440573758527371739379674409065046347677707672119140625;0.3542100117631397093731493441737256944179534912109375;-0.00799367136205268898063724947178343427367508411407470703125;0.038162084808005918012963064711584593169391155242919921875;-0.01068970617272657457064166663940341095440089702606201171875;-0.1330388415255171208340101429712376557290554046630859375;0.04684500486990676726417603958907420746982097625732421875;0.1943522227038603222837309658643789589405059814453125]
      mask Display: e = 0.06;c1 = [120 150 230]/255;c2 = ([120 150 230]+0)/383;c3 = ([120 150 230]+128)/383;patch([0 1 1 0],[0 0 1 1],c1);patch([0 1 1 1-e 1-e 0+e],[0 0 1 1-e 0+e 0+e],c2);patch([0 0 1 1-e 0+e 0+e],[0 1 1 1-e 1-e 0+e],c3);plot([0 1 1 0 0],[0 0 1 1 0]);disp('Weights');
  "IW{1,1}(50,:)'" : Constant  Value=[0.129238685931483299196287362065049819648265838623046875;-0.0269065670702432306604645617653659428469836711883544921875;-0.39392622767324814159195511820144020020961761474609375;0.35054492426896433077132542166509665548801422119140625;0.01144593719825746404306077153023579739965498447418212890625;-0.168010917126691250444991965196095407009124755859375;-0.05334374370762169637050220671881106682121753692626953125;0.09435278079493090996887616483945748768746852874755859375;0.1735366930304763910530851944713504053652286529541015625]
      mask Display: e = 0.06;c1 = [120 150 230]/255;c2 = ([120 150 230]+0)/383;c3 = ([120 150 230]+128)/383;patch([0 1 1 0],[0 0 1 1],c1);patch([0 1 1 1-e 1-e 0+e],[0 0 1 1-e 0+e 0+e],c2);patch([0 0 1 1-e 0+e 0+e],[0 1 1 1-e 1-e 0+e],c3);plot([0 1 1 0 0],[0 0 1 1 0]);disp('Weights');
  "IW{1,1}(6,:)'" : Constant  Value=[-0.2190476919951057366287017202921560965478420257568359375;-0.030812339510955751020748749624544871039688587188720703125;0.147184061221607820346690687074442394077777862548828125;0.2151847421857631947883504608398652635514736175537109375;-0.0673931697635940241131180528100230731070041656494140625;1.6392292042263674201052481294027529656887054443359375;-0.432734581803303708369412561296485364437103271484375;-0.2243165661088347972995649115546257235109806060791015625;-0.1730173543265577096317286986959516070783138275146484375]
      mask Display: e = 0.06;c1 = [120 150 230]/255;c2 = ([120 150 230]+0)/383;c3 = ([120 150 230]+128)/383;patch([0 1 1 0],[0 0 1 1],c1);patch([0 1 1 1-e 1-e 0+e],[0 0 1 1-e 0+e 0+e],c2);patch([0 0 1 1-e 0+e 0+e],[0 1 1 1-e 1-e 0+e],c3);plot([0 1 1 0 0],[0 0 1 1 0]);disp('Weights');
  "IW{1,1}(7,:)'" : Constant  Value=[-0.10198515251860397479166664425065391696989536285400390625;0.39081793692260047290432112276903353631496429443359375;-0.0895695319271929968341083849736605770885944366455078125;-0.01868304933144772361774954561042250134050846099853515625;0.000355927601077458554031107684778589828056283295154571533203125;0.040668261598205364404368111763687920756638050079345703125;0.1136040328493967688228138968042912892997264862060546875;-0.051293749084633633028573740375577472150325775146484375;-0.0384303676383060122123680457661976106464862823486328125]
      mask Display: e = 0.06;c1 = [120 150 230]/255;c2 = ([120 150 230]+0)/383;c3 = ([120 150 230]+128)/383;patch([0 1 1 0],[0 0 1 1],c1);patch([0 1 1 1-e 1-e 0+e],[0 0 1 1-e 0+e 0+e],c2);patch([0 0 1 1-e 0+e 0+e],[0 1 1 1-e 1-e 0+e],c3);plot([0 1 1 0 0],[0 0 1 1 0]);disp('Weights');
  "IW{1,1}(8,:)'" : Constant  Value=[-0.190570303261492990376524403473013080656528472900390625;-0.17333128135433006900001373651321046054363250732421875;0.732148322708408461068074757349677383899688720703125;-0.1565553064267309057999710830699768848717212677001953125;-0.280886551958949015617150735124596394598484039306640625;0.099473466131970333936607175928656943142414093017578125;0.0599996875288303643802834130838164128363132476806640625;-0.568258534666149284220182380522601306438446044921875;0.05074720405541287282513707168618566356599330902099609375]
      mask Display: e = 0.06;c1 = [120 150 230]/255;c2 = ([120 150 230]+0)/383;c3 = ([120 150 230]+128)/383;patch([0 1 1 0],[0 0 1 1],c1);patch([0 1 1 1-e 1-e 0+e],[0 0 1 1-e 0+e 0+e],c2);patch([0 0 1 1-e 0+e 0+e],[0 1 1 1-e 1-e 0+e],c3);plot([0 1 1 0 0],[0 0 1 1 0]);disp('Weights');
  "IW{1,1}(9,:)'" : Constant  Value=[0.35848984269573069827430344957974739372730255126953125;-0.50431229501068475240543875770526938140392303466796875;0.918400779092727770347437399323098361492156982421875;0.1797336157749873375433224964581313543021678924560546875;-0.375103362343016055735489544531446881592273712158203125;0.207054104960666729429163979148142971098423004150390625;0.01219111205402431154232179011387415812350809574127197265625;-0.0260723123346293418622909854320823797024786472320556640625;-0.07511421003692252129635420487829833291471004486083984375]
      mask Display: e = 0.06;c1 = [120 150 230]/255;c2 = ([120 150 230]+0)/383;c3 = ([120 150 230]+128)/383;patch([0 1 1 0],[0 0 1 1],c1);patch([0 1 1 1-e 1-e 0+e],[0 0 1 1-e 0+e 0+e],c2);patch([0 0 1 1-e 0+e 0+e],[0 1 1 1-e 1-e 0+e],c3);plot([0 1 1 0 0],[0 0 1 1 0]);disp('Weights');
  Mux : Mux  Inputs=50
      mask Display: e = 0.06;c1 = [120 150 230]/255;c2 = ([120 150 230]+0)/383;c3 = ([120 150 230]+128)/383;patch([0 1 1 0],[0 0 1 1],c1);patch([0 1 1 1-e 1-e 0+e],[0 0 1 1-e 0+e 0+e],c2);patch([0 0 1 1-e 0+e 0+e],[0 1 1 1-e 1-e 0+e],c3);plot([0 1 1 0 0],[0 0 1 1 0]);disp('Mux');
  dotprod{1..50} (50 alike) : neural/Weight Functions/dotprod
  "iz{1,1}" : Outport
      mask Display: e = 0.06;c1 = [120 230 180]/255;c2 = ([120 230 180]+0)/(256+128);c3 = ([120 230 180]+128)/(256+128);patch([0 1 1 0],[0 0 1 1],c1);patch([0 1 1 1-e 1-e 0+e],[0 0 1 1-e 0+e 0+e],c2);patch([0 0 1 1-e 0+e 0+e],[0 1 1 1-e 1-e 0+e],c3);plot([0 1 1 0 0],[0 0 1 1 0]);
  wires:
  "IW{1,1}(1,:)'"/1 -> dotprod1/1
  "pd{1,1}"/1 -> dotprod1/2, dotprod2/2, dotprod3/2, dotprod4/2, dotprod5/2, dotprod6/2, dotprod7/2, dotprod8/2, dotprod9/2, dotprod10/2, dotprod11/2, dotprod12/2, dotprod13/2, dotprod14/2, dotprod15/2, dotprod16/2, dotprod17/2, dotprod18/2, dotprod19/2, dotprod20/2, dotprod21/2, dotprod22/2, dotprod23/2, dotprod24/2, dotprod25/2, dotprod26/2, dotprod27/2, dotprod28/2, dotprod29/2, dotprod30/2, dotprod31/2, dotprod32/2, dotprod33/2, dotprod34/2, dotprod35/2, dotprod36/2, dotprod37/2, dotprod38/2, dotprod39/2, dotprod40/2, dotprod41/2, dotprod42/2, dotprod43/2, dotprod44/2, dotprod45/2, dotprod46/2, dotprod47/2, dotprod48/2, dotprod49/2, dotprod50/2
  dotprod1/1 -> Mux/1
  "IW{1,1}(2,:)'"/1 -> dotprod2/1
  dotprod2/1 -> Mux/2
  "IW{1,1}(3,:)'"/1 -> dotprod3/1
  dotprod3/1 -> Mux/3
  "IW{1,1}(4,:)'"/1 -> dotprod4/1
  dotprod4/1 -> Mux/4
  "IW{1,1}(5,:)'"/1 -> dotprod5/1
  dotprod5/1 -> Mux/5
  "IW{1,1}(6,:)'"/1 -> dotprod6/1
  dotprod6/1 -> Mux/6
  "IW{1,1}(7,:)'"/1 -> dotprod7/1
  dotprod7/1 -> Mux/7
  "IW{1,1}(8,:)'"/1 -> dotprod8/1
  dotprod8/1 -> Mux/8
  "IW{1,1}(9,:)'"/1 -> dotprod9/1
  dotprod9/1 -> Mux/9
  "IW{1,1}(10,:)'"/1 -> dotprod10/1
  dotprod10/1 -> Mux/10
  "IW{1,1}(11,:)'"/1 -> dotprod11/1
  dotprod11/1 -> Mux/11
  "IW{1,1}(12,:)'"/1 -> dotprod12/1
  dotprod12/1 -> Mux/12
  "IW{1,1}(13,:)'"/1 -> dotprod13/1
  dotprod13/1 -> Mux/13
  "IW{1,1}(14,:)'"/1 -> dotprod14/1
  dotprod14/1 -> Mux/14
  "IW{1,1}(15,:)'"/1 -> dotprod15/1
  dotprod15/1 -> Mux/15
  "IW{1,1}(16,:)'"/1 -> dotprod16/1
  dotprod16/1 -> Mux/16
  "IW{1,1}(17,:)'"/1 -> dotprod17/1
  dotprod17/1 -> Mux/17
  "IW{1,1}(18,:)'"/1 -> dotprod18/1
  dotprod18/1 -> Mux/18
  "IW{1,1}(19,:)'"/1 -> dotprod19/1
  dotprod19/1 -> Mux/19
  "IW{1,1}(20,:)'"/1 -> dotprod20/1
  dotprod20/1 -> Mux/20
  "IW{1,1}(21,:)'"/1 -> dotprod21/1
  dotprod21/1 -> Mux/21
  "IW{1,1}(22,:)'"/1 -> dotprod22/1
  dotprod22/1 -> Mux/22
  "IW{1,1}(23,:)'"/1 -> dotprod23/1
  dotprod23/1 -> Mux/23
  "IW{1,1}(24,:)'"/1 -> dotprod24/1
  dotprod24/1 -> Mux/24
  "IW{1,1}(25,:)'"/1 -> dotprod25/1
  dotprod25/1 -> Mux/25
  "IW{1,1}(26,:)'"/1 -> dotprod26/1
  dotprod26/1 -> Mux/26
  "IW{1,1}(27,:)'"/1 -> dotprod27/1
  dotprod27/1 -> Mux/27
  "IW{1,1}(28,:)'"/1 -> dotprod28/1
  dotprod28/1 -> Mux/28
  "IW{1,1}(29,:)'"/1 -> dotprod29/1
  dotprod29/1 -> Mux/29
  "IW{1,1}(30,:)'"/1 -> dotprod30/1
  dotprod30/1 -> Mux/30
  "IW{1,1}(31,:)'"/1 -> dotprod31/1
  dotprod31/1 -> Mux/31
  "IW{1,1}(32,:)'"/1 -> dotprod32/1
  dotprod32/1 -> Mux/32
  "IW{1,1}(33,:)'"/1 -> dotprod33/1
  dotprod33/1 -> Mux/33
  "IW{1,1}(34,:)'"/1 -> dotprod34/1
  dotprod34/1 -> Mux/34
  "IW{1,1}(35,:)'"/1 -> dotprod35/1
  dotprod35/1 -> Mux/35
  "IW{1,1}(36,:)'"/1 -> dotprod36/1
  dotprod36/1 -> Mux/36
  "IW{1,1}(37,:)'"/1 -> dotprod37/1
  dotprod37/1 -> Mux/37
  "IW{1,1}(38,:)'"/1 -> dotprod38/1
  dotprod38/1 -> Mux/38
  "IW{1,1}(39,:)'"/1 -> dotprod39/1
  dotprod39/1 -> Mux/39
  "IW{1,1}(40,:)'"/1 -> dotprod40/1
  dotprod40/1 -> Mux/40
  "IW{1,1}(41,:)'"/1 -> dotprod41/1
  dotprod41/1 -> Mux/41
  "IW{1,1}(42,:)'"/1 -> dotprod42/1
  dotprod42/1 -> Mux/42
  "IW{1,1}(43,:)'"/1 -> dotprod43/1
  dotprod43/1 -> Mux/43
  "IW{1,1}(44,:)'"/1 -> dotprod44/1
  dotprod44/1 -> Mux/44
  "IW{1,1}(45,:)'"/1 -> dotprod45/1
  dotprod45/1 -> Mux/45
  "IW{1,1}(46,:)'"/1 -> dotprod46/1
  dotprod46/1 -> Mux/46
  "IW{1,1}(47,:)'"/1 -> dotprod47/1
  dotprod47/1 -> Mux/47
  "IW{1,1}(48,:)'"/1 -> dotprod48/1
  dotprod48/1 -> Mux/48
  "IW{1,1}(49,:)'"/1 -> dotprod49/1
  dotprod49/1 -> Mux/49
  "IW{1,1}(50,:)'"/1 -> dotprod50/1
  dotprod50/1 -> Mux/50
  Mux/1 -> "iz{1,1}"/1
